simulink model "artificialPancreasWithFISTreeControl"  (R2022b)
settings: Solver=ode45  StartTime=0.0  StopTime=84600  MaxStep=100  RelTol=1e-6  EnableMultiTasking=on
PostLoadFcn:
  | load warmStart
  | Weight = 70;
  | Ts = 300;
  | closeLoop = 0;
undefined symbols (not defined in the file): fisT, warmStart
libraries: fuzblock x2, simulink x1
settings Model: Creator=The MathWorks, Inc.  LastModifiedBy=rajibhuq
settings SolverCC: AlgebraicLoopSolver=TrustRegion  MaxZcPerStep=1
settings DataIOCC: LimitDataPoints=on  SaveFormat=StructureWithTime
settings OptimizationCC: ExpressionDepthLimit=2147483647  LifeSpan=2  EfficientTunableParamExpr=on
settings DebuggingCC: SignalInfNanChecking=error  UnderspecifiedInitializationDetection=Classic  MergeDetectMultiDrivingBlocksExec=none  SolverPrmCheckMsg=warning  FcnCallInpInsideContextMsg=warning  UnconnectedInputMsg=warning  UnconnectedOutputMsg=warning  UnconnectedLineMsg=warning  BusObjectLabelMismatch=error  StateNameClashWarn=warning  SFUnexpectedBacktrackingDiag=warning  SFNoUnconditionalDefaultTransitionDiag=warning  SFExecutionAtInitializationDiag=none  SFMachineParentedDataDiag=warning  ArithmeticOperatorsInVariantConditions=warning
settings HardwareCC: ProdBitPerPointer=32  ProdBitPerSizeT=32  ProdBitPerPtrDiffT=32  ProdLargestAtomicFloat=None  ProdIntDivRoundTo=Undefined  ProdEndianess=Unspecified  ProdWordSize=32  ProdHWDeviceType=32-bit Generic
settings ModelReferenceCC: EnableRefExpFcnMdlSchedulingChecks=on  PropagateSignalLabelsOutOfModel=off
settings SFSimCC: SimUseLocalCustomCode=off  SimParseCustomCode=off  MATLABDynamicMemAlloc=off  CustomCodeUndefinedFunction=UseInterfaceOnly
settings RTWCC: Description=Create Visual C/C++ Solution File for the Real-Time Workshop Embedded Coder  SystemTargetFile=ert.tlc  PlatformDefinition=Embedded Code  TemplateMakefile=RTW.MSVCBuild  GenerateReport=on  RTWUseLocalCustomCode=off  IncludeHyperlinkInReport=on  LaunchReport=on  GenerateTraceInfo=on  GenerateTraceReport=on  GenerateTraceReportSl=on  GenerateTraceReportSf=on  GenerateTraceReportEml=on  DLArmComputeVersion=19.05
settings CodeAppCC: IgnoreCustomStorageClasses=off  CustomSymbolStrType=$N$R$M  StateflowObjectComments=on  InternalIdentifier=Classic
settings ERTTargetCC: MultiwordLength=2048  GenerateSampleERTMain=on  ERTCustomFileTemplate=example_file_process.tlc  ConvertIfToSwitch=off  SuppressUnreachableDefaultCases=off
settings ConfigComp: CovScope=Subsystem  CovPath=Sensor/Transducer/Transducer/Supervisory  CovMetricSettings=dcwe  CovHTMLOptions=-aTS=1 -bRG=1 -bTC=1 -hTR=0 -nFC=0 -scm=1 -bcm=1 -xEv=0  CovReportOnPause=off  CovExternalEMLEnable=off  DVMaxProcessTime=600  DVAutomaticStubbing=off  DVModelCoverageObjectives=MCDC  DVMaxTestCaseSteps=500  DVTestSuiteOptimization=CombinedObjectives  DVDetectActiveLogic=on  DVDetectOutOfBounds=on  DVSaveHarnessModel=on  DVSaveReport=on  PLC_OutputDir=./plcsrc  PLC_TargetIDE=rslogix5000  PLC_GenerateTestbench=on  PLC_MultiTBSigbuilderTimeRange=off  PLC_FoldFBCallOutputVar=off  PLC_InlineEnumCastFunction=off

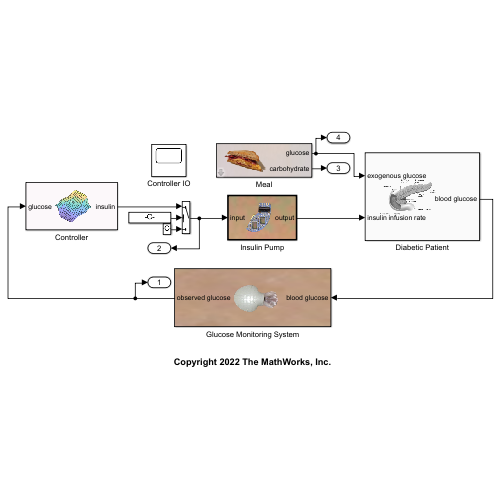
[thumbnail: Simulink's stored preview of the top-level diagram]
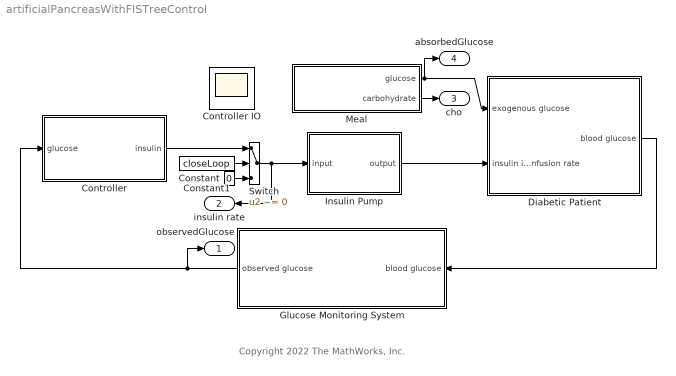
== system artificialPancreasWithFISTreeControl ==
  note: Copyright 2022 The MathWorks, Inc.
  Constant : Constant  Value=0
  Constant1 : Constant  Value=closeLoop
  Controller : Subsystem
      mask Display: image('$imagefile'); % Use "Edit Image" on toolstrip to change.
  Controller IO : Scope
      settings: Floating=on
  Diabetic Patient : Subsystem  RequirementInfo="{}  %GIDa_076720b2_3e47_4576_9667_7b10b7eaa38c"
      mask Display: image('$imagefile'); % Use "Edit Image" on toolstrip to change.
  Glucose Monitoring System : Subsystem
      mask Display: image('$imagefile'); % Use "Edit Image" on toolstrip to change.
  Insulin Pump : Subsystem  TreatAsAtomicUnit=on
      mask Display: image('$imagefile'); % Use "Edit Image" on toolstrip to change.
  Meal : Subsystem  mask{Ti=[60 300 720], DGu=[25 30 25], SMC=on, AG=0.8, tmaxG=40 * 60, allow=off}
      mask prompts: Ti "Starting Time Vector (min)"; DGu "CHO Amount Vector (g)"; SMC "Show model constants"; AG "CHO bioavailability (unitless)"; tmaxG "Time-to-maximum CHO absorption (sec)"; allow "Allow setting of additional output vector"
      mask help:
      | Parameters are vectors of the time each meal starts and the amount of carbohydrate in the meal.
      | Time unit is in minutes; CHO unit is in g, however, the output is in mmol, as used in the Hovorka model.
      | Block modifies model to generate additional output at the times of the meals plus a delta; without this the solver can miss some of the meals.
      mask init:
      | % Convert meal time to seconds.
      | Ti = Ti*60;
      | 
      | % Check for consistency of vector lengths
      | if (length(Ti)-length(DGu)),
      | 	error('Time and amount vectors must be of equal length');
      | end
      | 
      | % Model requires mmol
      | DG = DGu/0.18;
      | 
      | % Model parameters
      | delta = 1e-6;	% width of pulse for impulse
      | eavec = [0];
      | avec = [0];
      | tvec = [0];
      | for i = 1:length(Ti),
      | 	tvec = [tvec Ti(i) Ti(i) Ti(i)+delta Ti(i)+delta];
      | 	avec = [avec 0 DG(i)/delta DG(i)/delta 0];
      | 	eavec = [eavec 0 DGu(i)/delta DGu(i)/delta 0];
      | end
      | vecs = [tvec' avec'];
      | evecs = [tvec' eavec'];
      mask Callback SMC:
      | p = get_param(gcb,'MaskVisibilities');
      | if strcmp(get_param(gcb,'SMC'),'on'),
      | 	p(5) = {'on'};
      | 	p(6) = {'on'};
      | else
      | 	p(5) = {'off'};
      | 	p(6) = {'off'};
      | end
      | set_param(gcb,'MaskVisibilities',p);
      mask Display: image('$imagefile'); % Use "Edit Image" on toolstrip to change.
  Switch : Switch  Criteria=u2 ~= 0  SaturateOnIntegerOverflow=off  InputSameDT=off
  observedGlucose : Outport
  insulin rate : Outport  Port=2
  cho : Outport  Port=3
  absorbedGlucose : Outport  Port=4
  wires:
  Meal/1(glucose) -> absorbedGlucose/1, Diabetic Patient/1(exogenous glucose)
  Diabetic Patient/1(blood glucose) -> Glucose Monitoring System/1(blood glucose)
  Glucose Monitoring System/1(observed glucose) -> Controller/1(glucose), observedGlucose/1
  Meal/2(carbohydrate) -> cho/1
  Constant/1 -> Switch/3
  Constant1/1 -> Switch/2
  Switch/1 -> insulin rate/1, Insulin Pump/1(input)
  Controller/1(insulin) -> Switch/1
  Insulin Pump/1(output) -> Diabetic Patient/2(insulin infusion rate)

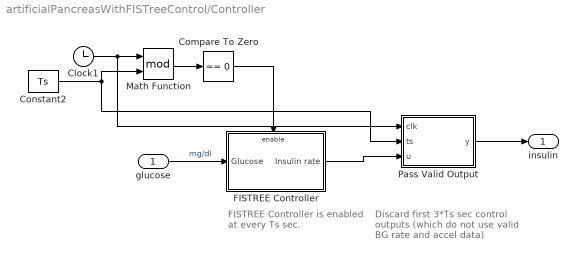
== system artificialPancreasWithFISTreeControl/Controller ==
  note: FISTREE Controller is enabled at every Ts sec.
  note: Discard first 3*Ts sec control outputs (which do not use valid BG rate and accel data)
  glucose : Inport
  Clock1 : Clock
  Compare To Zero : simulink/Logic and Bit Operations/Compare To Zero  relop===  OutDataTypeStr=boolean  ZeroCross=off
  Constant2 : Constant  Value=Ts
  FISTREE Controller : Subsystem  TreatAsAtomicUnit=on
  Math Function : Math  Operator=mod
  Pass Valid Output : MATLAB Function  TreatAsAtomicUnit=on
  insulin : Outport
  wires:
  Clock1/1 -> Pass Valid Output/1(clk), Math Function/1
  Pass Valid Output/1(y) -> insulin/1
  FISTREE Controller/1(Insulin rate) -> Pass Valid Output/3(u)
  Compare To Zero/1 -> FISTREE Controller/Enable
  Constant2/1 -> Pass Valid Output/2(ts), Math Function/2
  Math Function/1 -> Compare To Zero/1
  glucose/1 -> FISTREE Controller/1(Glucose)  "mg/dl"

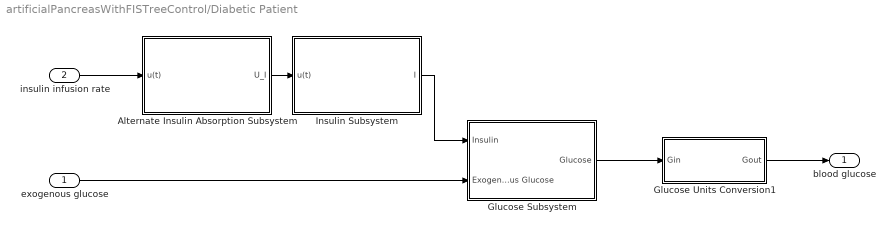
== system artificialPancreasWithFISTreeControl/Diabetic Patient ==
  exogenous glucose : Inport
  insulin infusion rate : Inport  Port=2
  Alternate Insulin Absorption Subsystem : Subsystem  mask{ka1=0.0112/60, ka2=0.0210/60, Vmaxld=1.93/60, kmld=62.6, k=0.67}
      mask prompts: ka1 "Slow channel transfer rate (1/sec)"; ka2 "Fast channel transfer rate (1/sec)"; Vmaxld "Saturation level V_{MAX,LD} (mU/sec)"; kmld "Half-concentration const. k_{M,LD} (mU)"; k "Proportion in slow channel"
      mask help:
      | Short-acting insulin infusion from subcutaneous injection (bolus or continuous), adapted from the selected model described in:
      | Wilinska et al. "Insulin kinetics in type-1 diabetes: continuous and bolus delivery of rapid acting insulin" IEEE Tran. Biomed. Eng. 52(1) 3-12, 2005.
      mask Help:
      | Short-acting insulin infusion from subcutaneous injection (bolus or continuous), adapted from the selected model described in:
      | Wilinska et al. "Insulin kinetics in type-1 diabetes: continuous and bolus delivery of rapid acting insulin" IEEE Tran. Biomed. Eng. 52(1) 3-12, 2005.
      | 
      | The only difference between the model as described in the paper and this implementation, is that only the absorption dynamics are preserved.  The dynamics of the plasma insulin compartment are eliminated, as the block of the original model can be used.
      | This gives us the term U_I(t) [using the notation of the original model]:
      | U_I(t) = k_{a1}Q_2 + k_{a2}Q_{1b }
      | which is the output of this block.
      | 
      | The 2005 paper indicates that the fractional clearance rate (k_e) and the insulin distribution volume (V_I) are not in the physiologic range when the model parameters are identified, but that the metabolic clearance rate (MRC = k_e*V_I) is.  This MRC is practically the same as that of the original model, thus the decision for the difference in implementation.
      | 
      | This model includes Michaelis-Menten saturation dynamics, and two absorption channels, one fast and one slow. Thus we need the additional parameters to describe the saturation behavior (V_{MAX,LD} and k_{M,LD}), and the constant k indicating the fraction of insulin going through the slow channel (leaving 1-k through the fast channel).
      mask Display:
      | port_label('input',1,'SC Ins Inf')
      | port_label('output',1,'Ins Abs Rate')
      | disp('Short-acting insulin\nsc infusion\n\n\nalternate')
  Glucose Subsystem : Subsystem  mask(Glucose Subsystem){SIT=(51.2e-4/2)/60, ISD=(8.2e-4/2)/60, SIE=(520e-4/2)/60, EGP0u=(0.0161)/60, F01u=(0.0097)/60, W=Weight, SMC=on, ka1=(0.006)/60, ka2=(0.06)/60, ka3=(0.03)/60, k12=(0.066)/60, VGu=0.16}
      mask prompts: SIT "Insulin sensitivity of distribution/transport (1/sec per mU/L)"; ISD "Insulin sensitivity of disposal (1/sec per mU/L)"; SIE "Insulin sensitivity of EGP (per mU/L)"; EGP0u "EGP @ zero insulin (mmol/(kg sec))"; F01u "Non-insulin-dependent glucose flux (mmol/(kg sec))"; W "Weight (kg)"; SMC "Show model constants"; ka1 "Deactivation rate ka1 (1/sec)"; ka2 "Deactivation rate ka2 (1/sec)"; ka3 "Deactivation rate ka3 (1/sec)"; k12 "Transfer rate k12 (1/sec)"; VGu "Glucose distribution volume (L/kg)"
      mask help:
      | This block describes the glucose and insulin effects on glucose as described in
      | Hovorka et al.
      mask init:
      | % Deactivation rates of insulin action on glucose
      | kb1 = ka1*SIT;
      | kb2 = ka2*ISD;
      | kb3 = ka3*SIE;
      | % Glucose distribution volume
      | VG = VGu*W; % [L/kg]*[kg]
      | % and also scale by weight
      | EGP0 = EGP0u*W;
      | F01 = F01u*W;
      mask Callback SMC:
      | p = get_param(gcb,'MaskVisibilities');
      | if strcmp(get_param(gcb,'SMC'),'on'),
      | 	p(8) = {'on'};
      | 	p(9) = {'on'};
      | 	p(10) = {'on'};
      | 	p(11) = {'on'};
      | 	p(12) = {'on'};
      | else
      | 	p(8) = {'off'};
      | 	p(9) = {'off'};
      | 	p(10) = {'off'};
      | 	p(11) = {'off'};
      | 	p(12) = {'off'};
      | end
      | set_param(gcb,'MaskVisibilities',p);
      mask Display:
      | port_label('input',1,'insulin')
      | port_label('input',2,'Exog. Gluc.')
      | port_label('output',1,'glucose')
      | disp('Glucose\n\n\n\n\nSubsystem')
  Glucose Units Conversion1 : Subsystem  mask{CNV=mM --> mg/dl}
      mask prompts: CNV "Glucose unit conversion"
      mask init:
      | switch CNV
      | 	case 1	% mM -> mg/dl
      | 		CF = 18;
      | 		txtin = 'mM';
      | 		txtout = 'mg/dl';
      | 	case 2	% mg/dl -> mM
      | 		CF = 1/18;
      | 		txtin = 'mg/dl';
      | 		txtout = 'mM';
      | end
      | 
      | set_param(gcb,'MaskDisplay',['port_label(''input'',1,txtin)' char(10) 'port_label(''output'',1,txtout)' char(10) 'disp(''Glucose\nUnits\nConversion'')'])
      mask TypeOptions CNV: mM --> mg/dl | mg/dl --> mM
      mask Display:
      | port_label('input',1,txtin)
      | port_label('output',1,txtout)
      | disp('Glucose\nUnits\nConversion')
  Insulin Subsystem : Subsystem  mask{W=Weight, SMC=off, VIu=0.12, ke=(0.138)/60}
      mask prompts: W "Weight (kg)"; SMC "Show model constants"; VIu "Insulin distribution volume (L/kg)"; ke "Insulin elimination from plasma (1/sec)"
      mask help:
      | Short-acting insulin infusion from subcutaneous injection (bolus or continuous), as described in:
      | Hovorka et al. "Nonlinear model predictive control of glucose concentration in subjects with type 1 diabetes" Physiol Meas 25 (2004) 905-920
      mask init:
      | % Insulin distribution volume
      | VI = VIu*W; % [L/kg]*[kg]
      | % Insulin elimination from plasma
      | %ke = 0.138; % 1/min
      mask Callback SMC:
      | p = get_param(gcb,'MaskVisibilities');
      | if strcmp(get_param(gcb,'SMC'),'on'),
      | 	p(3) = {'on'};
      | 	p(4) = {'on'};
      | else
      | 	p(3) = {'off'};
      | 	p(4) = {'off'};
      | end
      | set_param(gcb,'MaskVisibilities',p);
      mask Display:
      | port_label('input',1,'Ins Appr')
      | port_label('output',1,'Plasma Ins')
      | disp('Insulin\nSubsystem\n\n\n')
  blood glucose : Outport
  wires:
  Alternate Insulin Absorption Subsystem/1(U_I) -> Insulin Subsystem/1(u(t))
  Insulin Subsystem/1(I) -> Glucose Subsystem/1(Insulin)
  insulin infusion rate/1 -> Alternate Insulin Absorption Subsystem/1(u(t))
  exogenous glucose/1 -> Glucose Subsystem/2(Exogenous Glucose)
  Glucose Subsystem/1(Glucose) -> Glucose Units Conversion1/1(Gin)
  Glucose Units Conversion1/1(Gout) -> blood glucose/1

== system artificialPancreasWithFISTreeControl/Glucose Monitoring System ==
  blood glucose : Inport
  Zero-Order Hold : ZeroOrderHold  SampleTime=Ts
  observed glucose : Outport
  wires:
  Zero-Order Hold/1 -> observed glucose/1
  blood glucose/1 -> Zero-Order Hold/1

== system artificialPancreasWithFISTreeControl/Insulin Pump ==
  input : Inport
  output : Outport
  wires:
  input/1 -> output/1

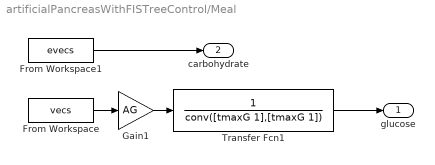
== system artificialPancreasWithFISTreeControl/Meal ==
  From Workspace : FromWorkspace  VariableName=vecs  OutputAfterFinalValue=Holding final value
  From Workspace1 : FromWorkspace  VariableName=evecs  OutputAfterFinalValue=Holding final value
  Gain1 : Gain  Gain=AG
  Transfer Fcn1 : TransferFcn  Denominator=conv([tmaxG 1],[tmaxG 1])
  glucose : Outport
  carbohydrate : Outport  Port=2
  wires:
  Transfer Fcn1/1 -> glucose/1
  From Workspace/1 -> Gain1/1
  Gain1/1 -> Transfer Fcn1/1
  From Workspace1/1 -> carbohydrate/1

== system artificialPancreasWithFISTreeControl/Controller/FISTREE Controller ==
  Glucose : Inport
  Enable : EnablePort
  Create BG Rates : Subsystem
  FISTREE : Subsystem
  Insulin rate : Outport
  wires:
  Glucose/1 -> Create BG Rates/1(BG_Level), FISTREE/1(BG_Level)  "mg/dl"
  FISTREE/1(out) -> Insulin rate/1
  Create BG Rates/1(BG_Rate) -> FISTREE/2(BG_Rate)  "mg/dl/min"
  Create BG Rates/2(BG_Accel) -> FISTREE/3(BG_Accel)  "mg/dl/min^2"

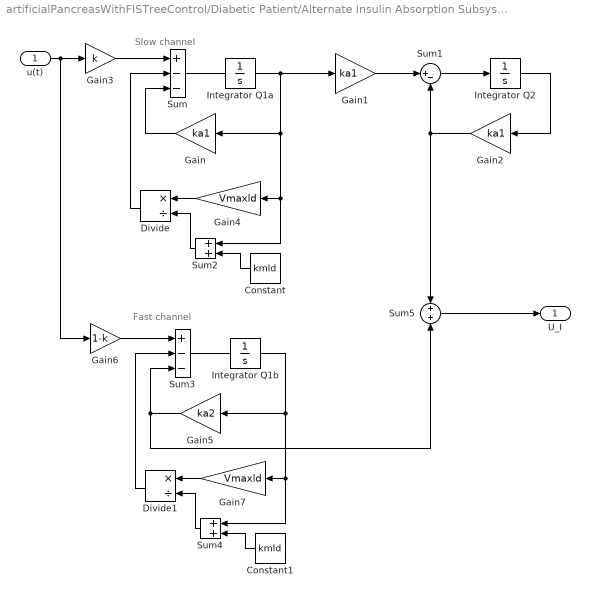
== system artificialPancreasWithFISTreeControl/Diabetic Patient/Alternate Insulin Absorption Subsystem ==
  note: Fast channel
  note: Slow channel
  u(t) : Inport
  Constant : Constant  Value=kmld
  Constant1 : Constant  Value=kmld
  Divide : Product  Inputs=*/
  Divide1 : Product  Inputs=*/
  Gain : Gain  Gain=ka1  SaturateOnIntegerOverflow=on  OutDataTypeStr=Inherit: Same as input  ParamDataTypeStr=Inherit: Same as input
  Gain1 : Gain  Gain=ka1  SaturateOnIntegerOverflow=on  OutDataTypeStr=Inherit: Same as input  ParamDataTypeStr=Inherit: Same as input
  Gain2 : Gain  Gain=ka1  SaturateOnIntegerOverflow=on  OutDataTypeStr=Inherit: Same as input  ParamDataTypeStr=Inherit: Same as input
  Gain3 : Gain  Gain=k
  Gain4 : Gain  Gain=Vmaxld  SaturateOnIntegerOverflow=on  OutDataTypeStr=Inherit: Same as input  ParamDataTypeStr=Inherit: Same as input
  Gain5 : Gain  Gain=ka2  SaturateOnIntegerOverflow=on  OutDataTypeStr=Inherit: Same as input  ParamDataTypeStr=Inherit: Same as input
  Gain6 : Gain  Gain=1-k
  Gain7 : Gain  Gain=Vmaxld  SaturateOnIntegerOverflow=on  OutDataTypeStr=Inherit: Same as input  ParamDataTypeStr=Inherit: Same as input
  Integrator Q1a : Integrator  InitialCondition=warmStart(3).values
  Integrator Q1b : Integrator  InitialCondition=warmStart(4).values
  Integrator Q2 : Integrator  InitialCondition=warmStart(5).values
  Sum : Sum  Inputs=+--  SaturateOnIntegerOverflow=on
  Sum1 : Sum  Inputs=|+-  SaturateOnIntegerOverflow=on
  Sum2 : Sum
  Sum3 : Sum  Inputs=+--  SaturateOnIntegerOverflow=on
  Sum4 : Sum
  Sum5 : Sum  Inputs=+|+
  U_I : Outport
  wires:
  Sum5/1 -> U_I/1
  Constant1/1 -> Sum4/2
  Sum4/1 -> Divide1/2
  Gain5/1 -> Sum5/2, Sum3/3
  Divide1/1 -> Sum3/2
  Gain7/1 -> Divide1/1
  Gain6/1 -> Sum3/1
  Sum3/1 -> Integrator Q1b/1
  Integrator Q1b/1 -> Sum4/1, Gain7/1, Gain5/1
  Integrator Q2/1 -> Gain2/1
  Gain2/1 -> Sum5/1, Sum1/2
  Sum1/1 -> Integrator Q2/1
  Gain1/1 -> Sum1/1
  Constant/1 -> Sum2/2
  Sum2/1 -> Divide/2
  Gain/1 -> Sum/3
  Divide/1 -> Sum/2
  Gain4/1 -> Divide/1
  Gain3/1 -> Sum/1
  u(t)/1 -> Gain6/1, Gain3/1
  Sum/1 -> Integrator Q1a/1
  Integrator Q1a/1 -> Gain1/1, Sum2/1, Gain4/1, Gain/1

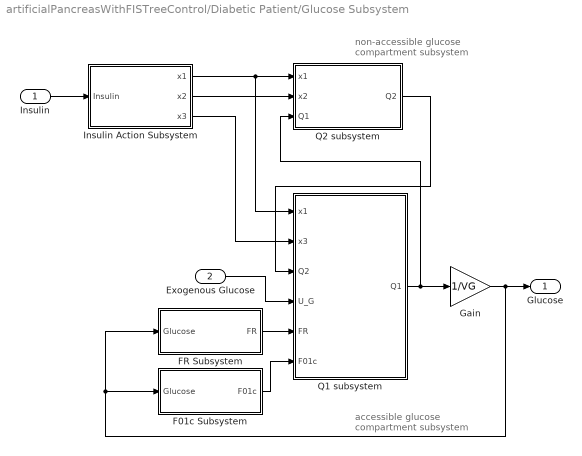
== system artificialPancreasWithFISTreeControl/Diabetic Patient/Glucose Subsystem ==
  note: accessible glucose
      | compartment subsystem
  note: non-accessible glucose
      | compartment subsystem
  Insulin : Inport
  Exogenous Glucose : Inport  Port=2
  F01c Subsystem : Subsystem
  FR Subsystem : Subsystem
  Gain : Gain  Gain=1/VG  SaturateOnIntegerOverflow=on  OutDataTypeStr=Inherit: Same as input  ParamDataTypeStr=Inherit: Same as input
  Insulin Action Subsystem : Subsystem
  Q1 subsystem : Subsystem
  Q2 subsystem : Subsystem
  Glucose : Outport
  wires:
  F01c Subsystem/1(F01c) -> Q1 subsystem/6(F01c)
  FR Subsystem/1(FR) -> Q1 subsystem/5(FR)
  Gain/1 -> F01c Subsystem/1(Glucose), FR Subsystem/1(Glucose), Glucose/1
  Insulin Action Subsystem/3(x3) -> Q1 subsystem/2(x3)
  Q1 subsystem/1(Q1) -> Gain/1, Q2 subsystem/3(Q1)
  Q2 subsystem/1(Q2) -> Q1 subsystem/3(Q2)
  Exogenous Glucose/1 -> Q1 subsystem/4(U_G)
  Insulin Action Subsystem/2(x2) -> Q2 subsystem/2(x2)
  Insulin Action Subsystem/1(x1) -> Q1 subsystem/1(x1), Q2 subsystem/1(x1)
  Insulin/1 -> Insulin Action Subsystem/1(Insulin)

== system artificialPancreasWithFISTreeControl/Diabetic Patient/Glucose Units Conversion1 ==
  Gin : Inport
  Conversion Factor : Gain  Gain=CF  SaturateOnIntegerOverflow=on  OutDataTypeStr=Inherit: Same as input  ParamDataTypeStr=Inherit: Same as input
  Gout : Outport
  wires:
  Conversion Factor/1 -> Gout/1
  Gin/1 -> Conversion Factor/1

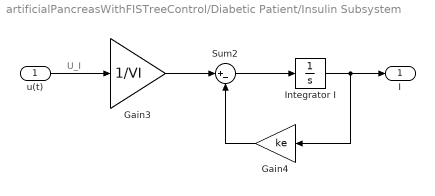
== system artificialPancreasWithFISTreeControl/Diabetic Patient/Insulin Subsystem ==
  note: U_I
  u(t) : Inport
  Gain3 : Gain  Gain=1/VI  SaturateOnIntegerOverflow=on  OutDataTypeStr=Inherit: Same as input  ParamDataTypeStr=Inherit: Same as input
  Gain4 : Gain  Gain=ke  SaturateOnIntegerOverflow=on  OutDataTypeStr=Inherit: Same as input  ParamDataTypeStr=Inherit: Same as input
  Integrator I : Integrator  InitialCondition=warmStart(2).values
  Sum2 : Sum  Inputs=|+-  SaturateOnIntegerOverflow=on
  I : Outport
  wires:
  Sum2/1 -> Integrator I/1
  Integrator I/1 -> I/1, Gain4/1
  Gain4/1 -> Sum2/2
  Gain3/1 -> Sum2/1
  u(t)/1 -> Gain3/1

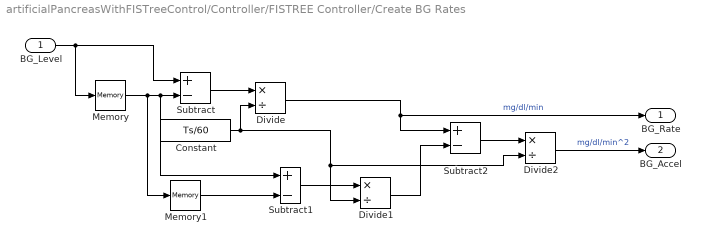
== system artificialPancreasWithFISTreeControl/Controller/FISTREE Controller/Create BG Rates ==
  BG_Level : Inport
  Constant : Constant  Value=Ts/60
  Divide : Product  Inputs=*/
  Divide1 : Product  Inputs=*/
  Divide2 : Product  Inputs=*/
  Memory : Memory  InheritSampleTime=on
  Memory1 : Memory  InheritSampleTime=on
  Subtract : Sum  Inputs=+-
  Subtract1 : Sum  Inputs=+-
  Subtract2 : Sum  Inputs=+-
  BG_Rate : Outport
  BG_Accel : Outport  Port=2
  wires:
  BG_Level/1 -> Subtract/1, Memory/1
  Subtract2/1 -> Divide2/1
  Memory/1 -> Memory1/1, Subtract/2, Subtract1/1
  Subtract1/1 -> Divide1/1
  Constant/1 -> Divide/2, Divide1/2, Divide2/2
  Divide2/1 -> BG_Accel/1  "mg/dl/min^2"
  Divide1/1 -> Subtract2/2
  Subtract/1 -> Divide/1
  Divide/1 -> BG_Rate/1, Subtract2/1  "mg/dl/min"
  Memory1/1 -> Subtract1/2

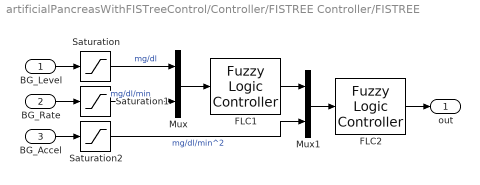
== system artificialPancreasWithFISTreeControl/Controller/FISTREE Controller/FISTREE ==
  BG_Level : Inport
  BG_Rate : Inport  Port=2
  BG_Accel : Inport  Port=3
  FLC1 : fuzblock/Fuzzy Logic  Controller  FIS=fisT.FIS(1)  OutputSampleNumber=101  DataType=double  FuzzifiedInputs=off  RuleFiringStrengths=off  RuleOutputs=off  AggregatedOutputs=off  SimulateUsing=Interpreted execution  OutOfRangeInputValueMessage=none  NoRuleFiredMessage=none  EmptyOutputFuzzySetMessage=none
  FLC2 : fuzblock/Fuzzy Logic  Controller  FIS=fisT.FIS(2)  OutputSampleNumber=101  DataType=double  FuzzifiedInputs=off  RuleFiringStrengths=off  RuleOutputs=off  AggregatedOutputs=off  SimulateUsing=Interpreted execution  OutOfRangeInputValueMessage=none  NoRuleFiredMessage=none  EmptyOutputFuzzySetMessage=none
  Mux : Mux  Inputs=2
  Mux1 : Mux  Inputs=2
  Saturation : Saturate  UpperLimit=fisT.FIS(1).Inputs(1).Range(2)  LowerLimit=fisT.FIS(1).Inputs(1).Range(1)  LinearizeAsGain=off  ZeroCross=off
  Saturation1 : Saturate  UpperLimit=fisT.FIS(1).Inputs(2).Range(2)  LowerLimit=fisT.FIS(1).Inputs(2).Range(1)  LinearizeAsGain=off  ZeroCross=off
  Saturation2 : Saturate  UpperLimit=fisT.FIS(2).Inputs(2).Range(2)  LowerLimit=fisT.FIS(2).Inputs(2).Range(1)  LinearizeAsGain=off  ZeroCross=off
  out : Outport
  wires:
  FLC1/1 -> Mux1/1
  BG_Rate/1 -> Saturation1/1
  BG_Level/1 -> Saturation/1
  Mux/1 -> FLC1/1
  Mux1/1 -> FLC2/1
  Saturation/1 -> Mux/1  "mg/dl"
  Saturation1/1 -> Mux/2  "mg/dl/min"
  Saturation2/1 -> Mux1/2  "mg/dl/min^2"
  FLC2/1 -> out/1
  BG_Accel/1 -> Saturation2/1

== system artificialPancreasWithFISTreeControl/Diabetic Patient/Glucose Subsystem/F01c Subsystem ==
  Glucose : Inport
  If : If  IfExpression=u1 >= 4.5
  If Action Subsystem : Subsystem  TreatAsAtomicUnit=on
  If Action Subsystem1 : Subsystem  TreatAsAtomicUnit=on
  Merge : Merge
  F01c : Outport
  wires:
  If Action Subsystem1/1(F01c) -> Merge/2
  If Action Subsystem/1(F01c) -> Merge/1
  Merge/1 -> F01c/1
  If/2 -> If Action Subsystem1/Action
  If/1 -> If Action Subsystem/Action
  Glucose/1 -> If Action Subsystem1/1(Glucose), If/1

== system artificialPancreasWithFISTreeControl/Diabetic Patient/Glucose Subsystem/FR Subsystem ==
  Glucose : Inport
  If : If  IfExpression=u1 < 9
  If Action Subsystem : Subsystem  TreatAsAtomicUnit=on
  If Action Subsystem1 : Subsystem  TreatAsAtomicUnit=on
  Merge : Merge
  FR : Outport
  wires:
  If Action Subsystem1/1(FR) -> Merge/2
  If Action Subsystem/1(Out1) -> Merge/1
  Merge/1 -> FR/1
  If/2 -> If Action Subsystem1/Action
  If/1 -> If Action Subsystem/Action
  Glucose/1 -> If Action Subsystem1/1(Glucose), If/1

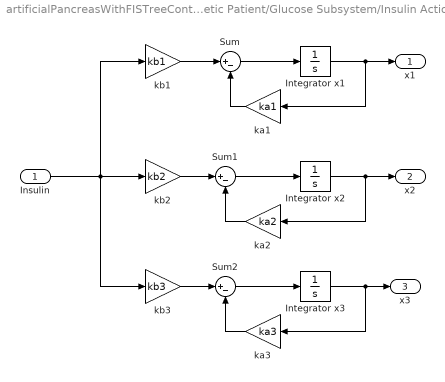
== system artificialPancreasWithFISTreeControl/Diabetic Patient/Glucose Subsystem/Insulin Action Subsystem ==
  Insulin : Inport
  Integrator x1 : Integrator  InitialCondition=warmStart(6).values
  Integrator x2 : Integrator  InitialCondition=warmStart(7).values
  Integrator x3 : Integrator  InitialCondition=warmStart(8).values
  Sum : Sum  Inputs=|+-  SaturateOnIntegerOverflow=on
  Sum1 : Sum  Inputs=|+-  SaturateOnIntegerOverflow=on
  Sum2 : Sum  Inputs=|+-  SaturateOnIntegerOverflow=on
  ka1 : Gain  Gain=ka1  SaturateOnIntegerOverflow=on  OutDataTypeStr=Inherit: Same as input  ParamDataTypeStr=Inherit: Same as input
  ka2 : Gain  Gain=ka2  SaturateOnIntegerOverflow=on  OutDataTypeStr=Inherit: Same as input  ParamDataTypeStr=Inherit: Same as input
  ka3 : Gain  Gain=ka3  SaturateOnIntegerOverflow=on  OutDataTypeStr=Inherit: Same as input  ParamDataTypeStr=Inherit: Same as input
  kb1 : Gain  Gain=kb1  SaturateOnIntegerOverflow=on  OutDataTypeStr=Inherit: Same as input  ParamDataTypeStr=Inherit: Same as input
  kb2 : Gain  Gain=kb2  SaturateOnIntegerOverflow=on  OutDataTypeStr=Inherit: Same as input  ParamDataTypeStr=Inherit: Same as input
  kb3 : Gain  Gain=kb3  SaturateOnIntegerOverflow=on  OutDataTypeStr=Inherit: Same as input  ParamDataTypeStr=Inherit: Same as input
  x1 : Outport
  x2 : Outport  Port=2
  x3 : Outport  Port=3
  wires:
  Integrator x3/1 -> x3/1, ka3/1
  Sum2/1 -> Integrator x3/1
  ka3/1 -> Sum2/2
  kb3/1 -> Sum2/1
  Integrator x2/1 -> x2/1, ka2/1
  Sum1/1 -> Integrator x2/1
  ka2/1 -> Sum1/2
  kb2/1 -> Sum1/1
  Integrator x1/1 -> x1/1, ka1/1
  Sum/1 -> Integrator x1/1
  ka1/1 -> Sum/2
  kb1/1 -> Sum/1
  Insulin/1 -> kb3/1, kb1/1, kb2/1

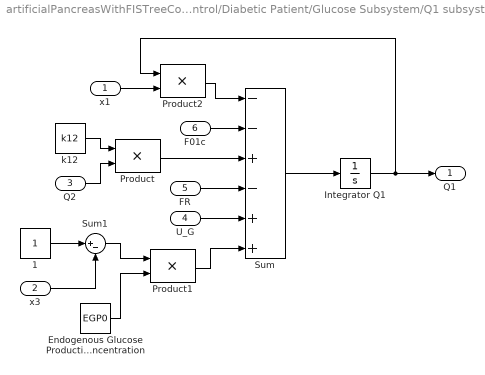
== system artificialPancreasWithFISTreeControl/Diabetic Patient/Glucose Subsystem/Q1 subsystem ==
  x1 : Inport
  x3 : Inport  Port=2
  Q2 : Inport  Port=3
  U_G : Inport  Port=4
  FR : Inport  Port=5
  F01c : Inport  Port=6
  1 : Constant
  Endogenous Glucose Production extrapolated to zero insulin concentration : Constant  Value=EGP0
  Integrator Q1 : Integrator  InitialCondition=warmStart(1).values
  Product : Product  SaturateOnIntegerOverflow=on  OutDataTypeStr=Inherit: Same as first input
  Product1 : Product  SaturateOnIntegerOverflow=on  OutDataTypeStr=Inherit: Same as first input
  Product2 : Product  SaturateOnIntegerOverflow=on  OutDataTypeStr=Inherit: Same as first input
  Sum : Sum  Inputs=--+-++  SaturateOnIntegerOverflow=on
  Sum1 : Sum  Inputs=|+-  SaturateOnIntegerOverflow=on
  k12 : Constant  Value=k12
  Q1 : Outport
  wires:
  F01c/1 -> Sum/2
  Product/1 -> Sum/3
  FR/1 -> Sum/4
  U_G/1 -> Sum/5
  Product1/1 -> Sum/6
  x1/1 -> Product2/2
  Product2/1 -> Sum/1
  Sum/1 -> Integrator Q1/1
  Endogenous Glucose Production extrapolated to zero insulin concentration/1 -> Product1/2
  Sum1/1 -> Product1/1
  x3/1 -> Sum1/2
  1/1 -> Sum1/1
  Q2/1 -> Product/2
  k12/1 -> Product/1
  Integrator Q1/1 -> Product2/1, Q1/1

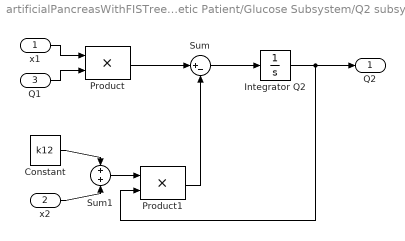
== system artificialPancreasWithFISTreeControl/Diabetic Patient/Glucose Subsystem/Q2 subsystem ==
  x1 : Inport
  x2 : Inport  Port=2
  Q1 : Inport  Port=3
  Constant : Constant  Value=k12
  Integrator Q2 : Integrator  InitialCondition=warmStart(9).values
  Product : Product  SaturateOnIntegerOverflow=on  OutDataTypeStr=Inherit: Same as first input
  Product1 : Product  SaturateOnIntegerOverflow=on  OutDataTypeStr=Inherit: Same as first input
  Sum : Sum  Inputs=|+-  SaturateOnIntegerOverflow=on
  Sum1 : Sum  Inputs=+|+  SaturateOnIntegerOverflow=on
  Q2 : Outport
  wires:
  Integrator Q2/1 -> Product1/2, Q2/1
  Sum/1 -> Integrator Q2/1
  Product1/1 -> Sum/2
  Sum1/1 -> Product1/1
  x2/1 -> Sum1/2
  Constant/1 -> Sum1/1
  Product/1 -> Sum/1
  Q1/1 -> Product/2
  x1/1 -> Product/1

== system artificialPancreasWithFISTreeControl/Diabetic Patient/Glucose Subsystem/F01c Subsystem/If Action Subsystem ==
  Action Port : ActionPort  ActionPortLabel=if(u1 >= 4.5)
  Constant : Constant  Value=F01
  F01c : Outport  InitialOutput=F01
  wires:
  Constant/1 -> F01c/1

== system artificialPancreasWithFISTreeControl/Diabetic Patient/Glucose Subsystem/F01c Subsystem/If Action Subsystem1 ==
  Glucose : Inport
  Action Port : ActionPort  ActionPortLabel=else
  Gain : Gain  Gain=F01/4.5  SaturateOnIntegerOverflow=on  OutDataTypeStr=Inherit: Same as input  ParamDataTypeStr=Inherit: Same as input
  F01c : Outport
  wires:
  Glucose/1 -> Gain/1
  Gain/1 -> F01c/1

== system artificialPancreasWithFISTreeControl/Diabetic Patient/Glucose Subsystem/FR Subsystem/If Action Subsystem ==
  Action Port : ActionPort  ActionPortLabel=if(u1 < 9)
  Constant : Constant  Value=0
  Out1 : Outport  InitialOutput=0
  wires:
  Constant/1 -> Out1/1

== system artificialPancreasWithFISTreeControl/Diabetic Patient/Glucose Subsystem/FR Subsystem/If Action Subsystem1 ==
  Glucose : Inport
  Action Port : ActionPort  ActionPortLabel=else
  Constant : Constant  Value=9
  Gain : Gain  Gain=0.003*VG/60  SaturateOnIntegerOverflow=on  OutDataTypeStr=Inherit: Same as input  ParamDataTypeStr=Inherit: Same as input
  Sum : Sum  Inputs=|+-  SaturateOnIntegerOverflow=on
  FR : Outport
  wires:
  Gain/1 -> FR/1
  Sum/1 -> Gain/1
  Constant/1 -> Sum/2
  Glucose/1 -> Sum/1

== matlab function artificialPancreasWithFISTreeControl/Controller/Pass Valid Output ==
  data: clk input; ts input; u input; y output
function y = fcn(clk,ts,u)

if clk < 3*ts
    y = 0;
else
    y = u;
end
